simulink model "Linear_Controller_Nonlinear_Plant"  (R2025b)
settings: Solver=VariableStepAuto  StartTime=0.0  StopTime=100.0  RelTol=1e-3
undefined symbols (not defined in the file or in its folder): K, p
settings Model: Creator=chako  LastModifiedBy=chako

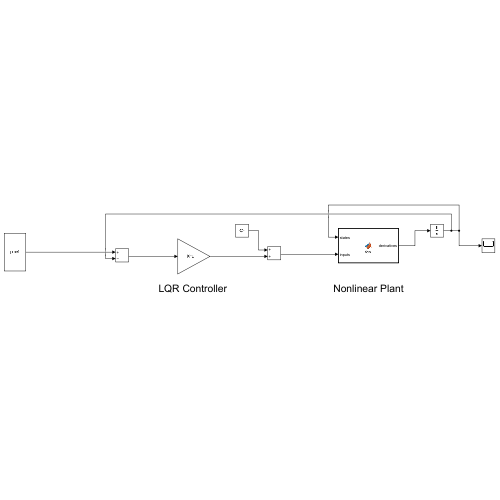
[thumbnail: Simulink's stored preview of the top-level diagram]
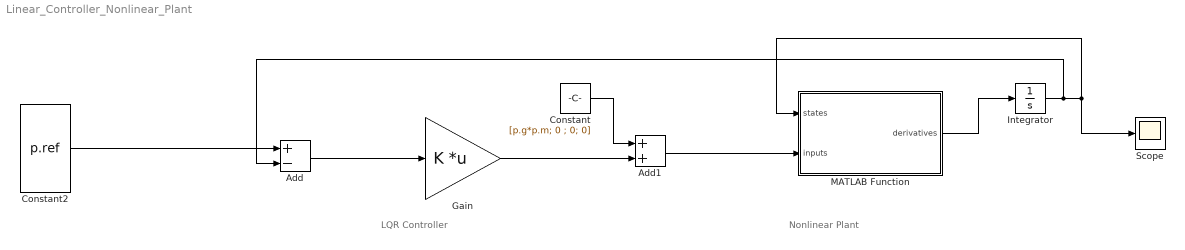
== system Linear_Controller_Nonlinear_Plant ==
  note: Nonlinear Plant
  note: LQR Controller
  Add : Sum  Inputs=+-
  Add1 : Sum
  Constant : Constant  Value=[p.g*p.m; 0 ; 0; 0]
  Constant2 : Constant  Value=p.ref
  Gain : Gain  Gain=K  Multiplication=Matrix(K*u)
  Integrator : Integrator  InitialCondition=[0;0;0;0;0;0;0;0;0;0;0;0]
  MATLAB Function : MATLAB Function  TreatAsAtomicUnit=on
  Scope : Scope
      settings: ActiveDisplayYMinimum=-2.9166662979596856  ActiveDisplayYMaximum=20.948446100131591
  wires:
  Integrator/1 -> Add/2, MATLAB Function/1(states), Scope/1
  Constant2/1 -> Add/1
  Add/1 -> Gain/1
  MATLAB Function/1(derivatives) -> Integrator/1
  Add1/1 -> MATLAB Function/2(inputs)
  Gain/1 -> Add1/2
  Constant/1 -> Add1/1

== matlab function Linear_Controller_Nonlinear_Plant/MATLAB Function ==
  data: states input size=12; derivatives output size=12; inputs input size=4; p parameter
function derivatives = fcn(states, inputs, p)

 % I is the inertia matrix
    I = [p.Ixx 0 0;
         0 p.Iyy 0;
         0 0 p.Izz];

    xi= states(1:3); % x, y, z
    xid = states(4:6); %x_prime, y_prime, z_prime
    eta = states(7:9); % roll, pitch, yaw
    etad = states(10:12); % roll_prime, pitch_prime, yaw_prime

    % Cosines of each
    c_roll = cos(eta(1));
    c_pitch = cos(eta(2));
    c_yaw = cos(eta(3));

    % Sines of each
    s_roll = sin(eta(1));
    s_pitch = sin(eta(2));
    s_yaw = sin(eta(3));


    % Derivative of xi is xid

    % Calculative derivatives of xid
    xidd = [0;0;-p.g] - (p.kD/p.m)*xid + ...
        ([s_roll*s_yaw + c_roll*s_pitch*c_yaw;
         c_roll*s_pitch*s_yaw - s_roll*c_yaw;
         c_roll*c_pitch]*inputs(1))*1/p.m; % Dividing by m here


    % Derivative of eta is etad
    % Calculative derivatives of etad


    % eta is [phi, theta, psi] = roll pitch yaw
    W = [1  0       -s_pitch;
         0  c_roll  s_roll * c_pitch;
         0 -s_roll  c_roll * c_pitch];
    % v is rpy in body frame
    
    tau_body = [inputs(2);
                inputs(3);
                inputs(4)];
    v = W * etad;
    vd = inv(I) * (tau_body + [(p.Iyy - p.Izz)*v(2)*v(3); ... 
                               (p.Izz - p.Ixx)*v(1)*v(3);
                               (p.Ixx - p.Iyy)*v(1)*v(2)]);
    Wd = [0        0                  -etad(2)*cos(-etad(2));
          0 -etad(1)*s_roll            etad(1)*c_roll*c_pitch;
          0 -etad(1)*c_roll -etad(1)*s_roll*c_pitch-etad(2)*c_roll*s_pitch];
    etadd = inv(W) * (vd - Wd*etad);
    derivatives = [xid; xidd; etad; etadd];
end
